simulink model "untitled"  (R2025b)
settings: Solver=VariableStepAuto  StartTime=0.0  StopTime=20  RelTol=1e-3
model workspace (MAT data in the model file):
  M = 1
settings Model: Creator=stand  LastModifiedBy=stand

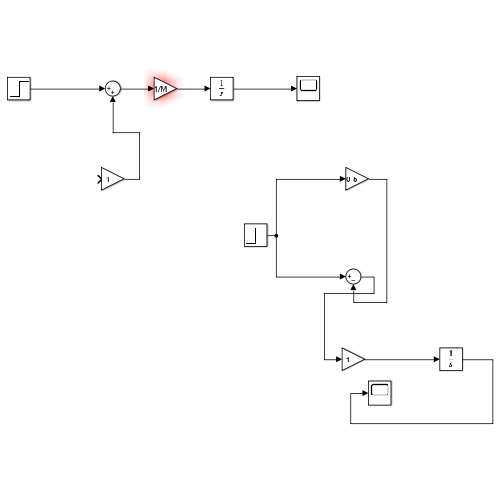
[thumbnail: Simulink's stored preview of the top-level diagram]
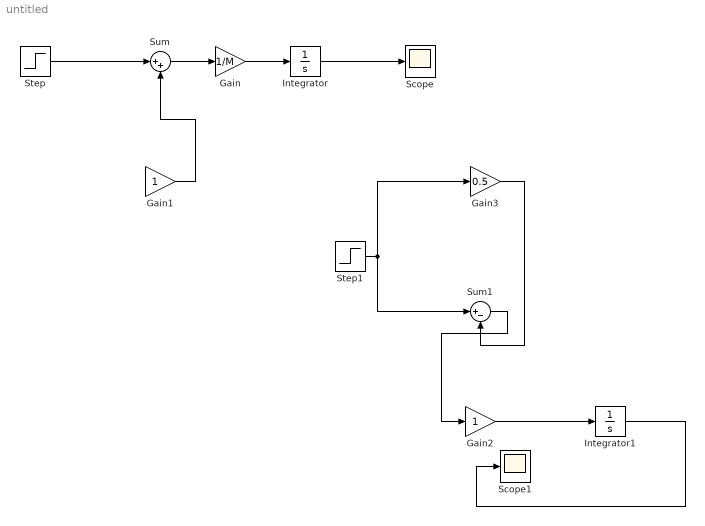
== system untitled ==
  Gain : Gain  Gain=1/M
  Gain1 : Gain
  Gain2 : Gain
  Gain3 : Gain  Gain=0.5
  Integrator : Integrator
  Integrator1 : Integrator
  Scope : Scope
  Scope1 : Scope
  Step : Step  SampleTime=0
  Step1 : Step  Time=0  SampleTime=0
  Sum : Sum  Inputs=|++
  Sum1 : Sum  Inputs=|+-
  wires:
  Step/1 -> Sum/1
  Integrator/1 -> Scope/1
  Gain/1 -> Integrator/1
  Sum/1 -> Gain/1
  Gain1/1 -> Sum/2
  Integrator1/1 -> Scope1/1
  Gain2/1 -> Integrator1/1
  Step1/1 -> Gain3/1, Sum1/1
  Gain3/1 -> Sum1/2
  Sum1/1 -> Gain2/1
